simulink model "EngineCoolingFanController"  (R2025a)
settings: Solver=VariableStepAuto  StartTime=0.0  StopTime=10.0  RelTol=1e-3
undefined symbols (not defined in the file or in its folder): cal_f32HystHalf, cal_f32TempHighLim, cal_f32TempThresh, cal_u8FanSpeedCmd
settings Model: Creator=wangtianqi  LastModifiedBy=wangtianqi

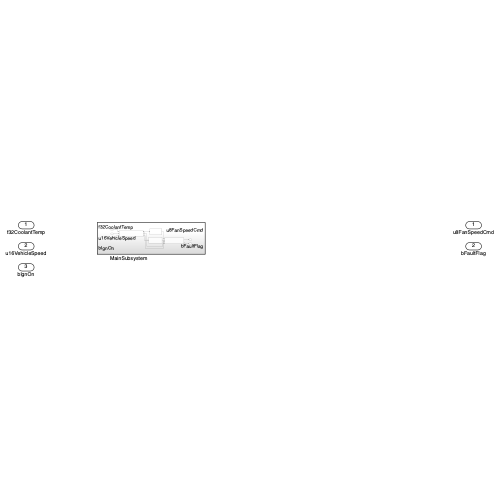
[thumbnail: Simulink's stored preview of the top-level diagram]
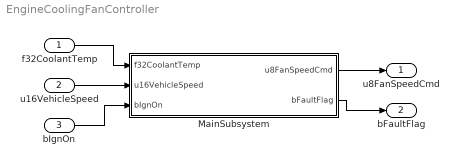
== system EngineCoolingFanController ==
  f32CoolantTemp : Inport  OutDataTypeStr=single
  u16VehicleSpeed : Inport  Port=2  OutDataTypeStr=uint16
  bIgnOn : Inport  Port=3  OutDataTypeStr=boolean
  MainSubsystem : Subsystem
  u8FanSpeedCmd : Outport  OutDataTypeStr=uint8
  bFaultFlag : Outport  Port=2  OutDataTypeStr=boolean
  wires:
  bIgnOn/1 -> MainSubsystem/3(bIgnOn)
  MainSubsystem/2(bFaultFlag) -> bFaultFlag/1
  MainSubsystem/1(u8FanSpeedCmd) -> u8FanSpeedCmd/1
  u16VehicleSpeed/1 -> MainSubsystem/2(u16VehicleSpeed)
  f32CoolantTemp/1 -> MainSubsystem/1(f32CoolantTemp)

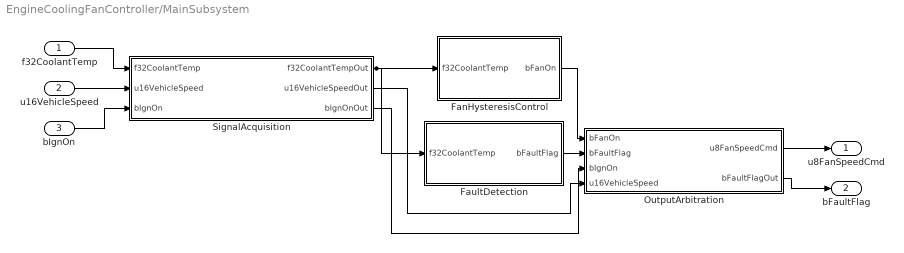
== system EngineCoolingFanController/MainSubsystem ==
  f32CoolantTemp : Inport  OutDataTypeStr=single
  u16VehicleSpeed : Inport  Port=2  OutDataTypeStr=uint16
  bIgnOn : Inport  Port=3  OutDataTypeStr=boolean
  FanHysteresisControl : Subsystem
  FaultDetection : Subsystem
  OutputArbitration : Subsystem
  SignalAcquisition : Subsystem
  u8FanSpeedCmd : Outport  OutDataTypeStr=uint8
  bFaultFlag : Outport  Port=2  OutDataTypeStr=boolean
  wires:
  FanHysteresisControl/1(bFanOn) -> OutputArbitration/1(bFanOn)
  SignalAcquisition/1(f32CoolantTempOut) -> FaultDetection/1(f32CoolantTemp), FanHysteresisControl/1(f32CoolantTemp)
  SignalAcquisition/2(u16VehicleSpeedOut) -> OutputArbitration/4(u16VehicleSpeed)
  bIgnOn/1 -> SignalAcquisition/3(bIgnOn)
  FaultDetection/1(bFaultFlag) -> OutputArbitration/2(bFaultFlag)
  SignalAcquisition/3(bIgnOnOut) -> OutputArbitration/3(bIgnOn)
  u16VehicleSpeed/1 -> SignalAcquisition/2(u16VehicleSpeed)
  OutputArbitration/2(bFaultFlagOut) -> bFaultFlag/1
  OutputArbitration/1(u8FanSpeedCmd) -> u8FanSpeedCmd/1
  f32CoolantTemp/1 -> SignalAcquisition/1(f32CoolantTemp)

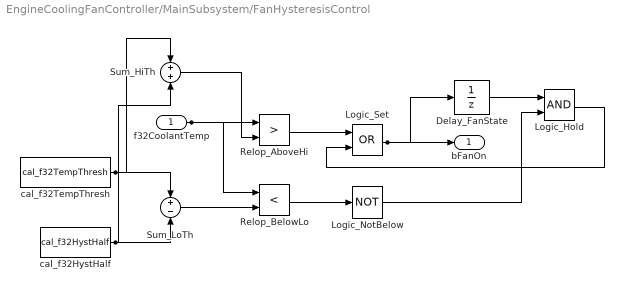
== system EngineCoolingFanController/MainSubsystem/FanHysteresisControl ==
  f32CoolantTemp : Inport
  Delay_FanState : UnitDelay  SampleTime=-1  HasFrameUpgradeWarning=on
  Logic_Hold : Logic  AllPortsSameDT=off  OutDataTypeStr=boolean
  Logic_NotBelow : Logic  Operator=NOT  Inputs=1  AllPortsSameDT=off  OutDataTypeStr=boolean
  Logic_Set : Logic  Operator=OR  AllPortsSameDT=off  OutDataTypeStr=boolean
  Relop_AboveHi : RelationalOperator  Operator=>  OutDataTypeStr=boolean  RndMeth=Simplest  InputSameDT=off
  Relop_BelowLo : RelationalOperator  Operator=<  OutDataTypeStr=boolean  RndMeth=Simplest  InputSameDT=off
  Sum_HiTh : Sum  OutDataTypeStr=single
  Sum_LoTh : Sum  Inputs=+-  OutDataTypeStr=single
  cal_f32HystHalf : Constant  Value=cal_f32HystHalf  OutDataTypeStr=single
  cal_f32TempThresh : Constant  Value=cal_f32TempThresh  OutDataTypeStr=single
  bFanOn : Outport
  wires:
  Logic_Hold/1 -> Logic_Set/2
  Delay_FanState/1 -> Logic_Hold/1
  Logic_NotBelow/1 -> Logic_Hold/2
  Logic_Set/1 -> Delay_FanState/1, bFanOn/1
  Relop_AboveHi/1 -> Logic_Set/1
  Sum_LoTh/1 -> Relop_BelowLo/2
  f32CoolantTemp/1 -> Relop_BelowLo/1, Relop_AboveHi/1
  cal_f32HystHalf/1 -> Sum_HiTh/2, Sum_LoTh/2
  Relop_BelowLo/1 -> Logic_NotBelow/1
  Sum_HiTh/1 -> Relop_AboveHi/2
  cal_f32TempThresh/1 -> Sum_LoTh/1, Sum_HiTh/1

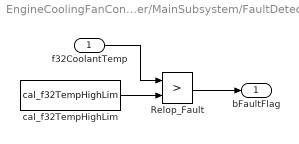
== system EngineCoolingFanController/MainSubsystem/FaultDetection ==
  f32CoolantTemp : Inport
  Relop_Fault : RelationalOperator  Operator=>  OutDataTypeStr=boolean  RndMeth=Simplest  InputSameDT=off
  cal_f32TempHighLim : Constant  Value=cal_f32TempHighLim  OutDataTypeStr=single
  bFaultFlag : Outport
  wires:
  Relop_Fault/1 -> bFaultFlag/1
  cal_f32TempHighLim/1 -> Relop_Fault/2
  f32CoolantTemp/1 -> Relop_Fault/1

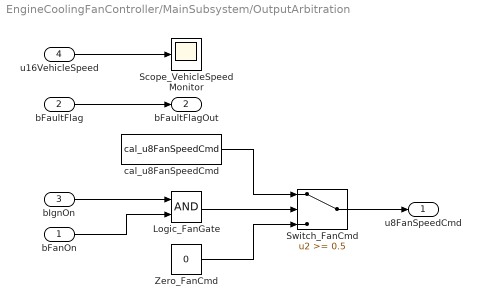
== system EngineCoolingFanController/MainSubsystem/OutputArbitration ==
  bFanOn : Inport
  bFaultFlag : Inport  Port=2
  bIgnOn : Inport  Port=3
  u16VehicleSpeed : Inport  Port=4
  Logic_FanGate : Logic  AllPortsSameDT=off  OutDataTypeStr=boolean
  Scope_VehicleSpeedMonitor : Scope
  Switch_FanCmd : Switch  Threshold=0.5  OutDataTypeStr=uint8  SaturateOnIntegerOverflow=off  InputSameDT=off
  Zero_FanCmd : Constant  Value=0  OutDataTypeStr=uint8
  cal_u8FanSpeedCmd : Constant  Value=cal_u8FanSpeedCmd  OutDataTypeStr=uint8
  u8FanSpeedCmd : Outport
  bFaultFlagOut : Outport  Port=2
  wires:
  Logic_FanGate/1 -> Switch_FanCmd/2
  Zero_FanCmd/1 -> Switch_FanCmd/3
  bFanOn/1 -> Logic_FanGate/2
  bIgnOn/1 -> Logic_FanGate/1
  Switch_FanCmd/1 -> u8FanSpeedCmd/1
  cal_u8FanSpeedCmd/1 -> Switch_FanCmd/1
  bFaultFlag/1 -> bFaultFlagOut/1
  u16VehicleSpeed/1 -> Scope_VehicleSpeedMonitor/1

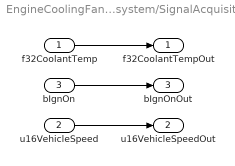
== system EngineCoolingFanController/MainSubsystem/SignalAcquisition ==
  f32CoolantTemp : Inport
  u16VehicleSpeed : Inport  Port=2
  bIgnOn : Inport  Port=3
  f32CoolantTempOut : Outport
  u16VehicleSpeedOut : Outport  Port=2
  bIgnOnOut : Outport  Port=3
  wires:
  u16VehicleSpeed/1 -> u16VehicleSpeedOut/1
  bIgnOn/1 -> bIgnOnOut/1
  f32CoolantTemp/1 -> f32CoolantTempOut/1
